simulink model "Model_5"  (R2020b)
settings: Solver=VariableStepAuto  StartTime=0.0  StopTime=10.0  RelTol=1e-3
settings Model: Creator=Akarsh  LastModifiedBy=Akarsh

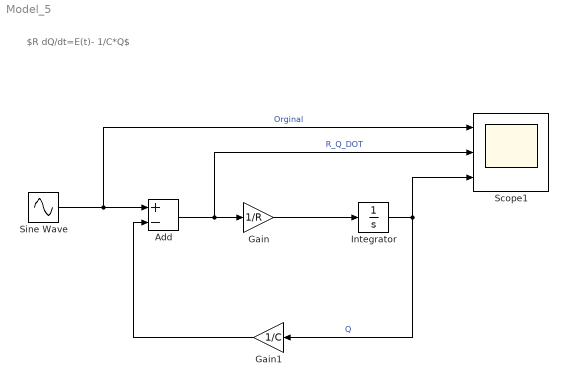
== system Model_5 ==
  note: $R dQ/dt=E(t)- 1/C*Q$
  Add : Sum  Inputs=+-
  Gain : Gain  Gain=1/R  mask{R=10}
  Gain1 : Gain  Gain=1/C  mask{C=10^-6}
  Integrator : Integrator
  Scope1 : Scope  NumInputPorts=3
  Sine Wave : Sin  SampleTime=0
  wires:
  Integrator/1 -> Gain1/1, Scope1/3  "Q"
  Sine Wave/1 -> Scope1/1, Add/1  "Orginal"
  Gain1/1 -> Add/2
  Add/1 -> Gain/1, Scope1/2  "R_Q_DOT"
  Gain/1 -> Integrator/1
